simulink model "TestPDURacks"  (R2025b)
settings: Solver=daessc  StartTime=0.0  StopTime=1200  MaxStep=1  RelTol=1e-3  AbsTol=1e-3
libraries: nesl_utility x5, fl_lib x4, datacenterCompositeLib x1
settings Model: Creator=vikrants  LastModifiedBy=vikrants
settings SolverCC: AutoScaleAbsTol=off  AlgebraicLoopSolver=TrustRegion  MaxZcPerStep=1.0
settings DebuggingCC: UnconnectedInputMsg=warning  UnconnectedOutputMsg=warning  UnconnectedLineMsg=warning  SymbolicDimsDataTypeCodeGenerationDiagnostic=none
settings ModelReferenceCC: EnableRefExpFcnMdlSchedulingChecks=on
settings SFSimCC: CustomCodeUndefinedFunction=UseInterfaceOnly
settings RTWCC: GPUComputeCapability=3.5  DLArmComputeVersion=19.05
settings SimscapeCC: SimscapeLogType=all  SimscapeLogSimulationStatistics=on  SimscapeLogDataHistory=10000.0

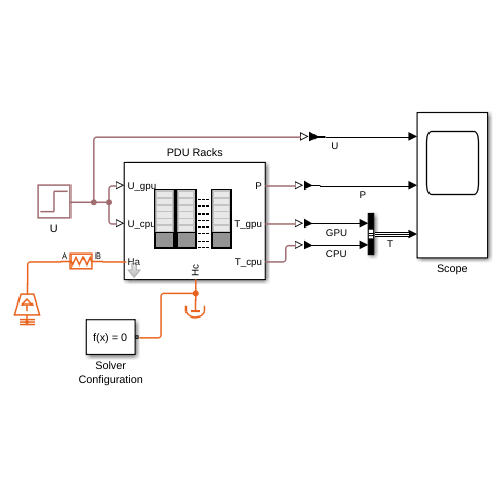
[thumbnail: Simulink's stored preview of the top-level diagram]
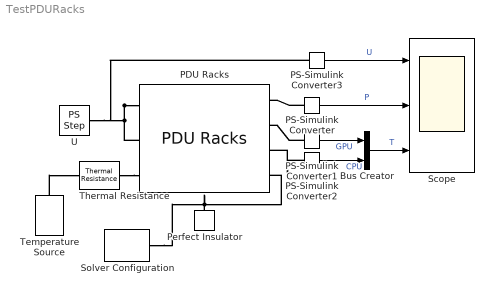
== system TestPDURacks ==
  Bus Creator : BusCreator  Inputs=2
  PDU Racks : datacenterCompositeLib/PDU Racks  nTrays=6  nRacks=4  trayMass=5  trayCp=2000  trayThermalR=0.1  nGPU=1  gpuTDPperDie=1200  gpuIdlePower=300  gpuHBMpower=80  gpuExponent=1.4  gpuHBMutil=0.7  gpuLeakage=1.5  gpuNominalDieT=350  gpuDieThermalC=50  gpuHeatSinkR=0.15  gpuSurfArea=0.01  gpuAmbientR=0.5  nCPU=1  cpuTDPperSocket=350  cpuIdlePower=80  cpuExponent=1.1  cpuLeakage=1.5  cpuNominalDieT=350  cpuDieThermalC=50  cpuHeatSinkR=0.15  cpuSurfArea=0.01  cpuAmbientR=0.5  initialT=350  htc=10
  PS-Simulink Converter{,1..3} (4 alike) : nesl_utility/PS-Simulink Converter  PhysicalDomain=network_engine_domain  SubClassName=ps_output  LeftPortType=input  RightPortType=output  PseudoPeriodic=off  Frequencies=[]  VectorFormat=inherit  Unit=inherit  AffineConversion=off
  Perfect Insulator : fl_lib/Thermal/Thermal Elements/Perfect Insulator  T_specify=off  T_priority=None  T=293.15 K  T_nominal_specify=off  T_nominal_value=1  T_nominal_unit=K
  Scope : Scope  NumInputPorts=3
      settings: ActiveDisplayYMinimum=0.15000000000000002  ActiveDisplayYMaximum=0.64999999999999991
  Solver Configuration : nesl_utility/Solver Configuration  PhysicalDomain=network_engine_domain  SubClassName=solver  LeftPortType=input  RightPortType=generic  Tones=[]  Harmonics=[]  SimulateNoise=off  Profile=off  UseLocalSampling=off  EnableSwitchedLinearOptims=on  FrequencyDomain=off  UseCCode=off  RelTol=0.001  AbsTol=1e-06  MinStep=1e-09  ToWorkspace=off  RevertToSquareIcSolve=off  NumHomotopyIterations=100  PhasorMode=off  PhasorModeNumHarmonics=1  ConsistencySolver=NEWTON_XTOL_AFTER_FTOL  IndexReductionMethod=DerivativeReplacement  DoDC=off  ResidualTolerance=1e-09  ConsistencyTolSource=GLOBAL  ConsistencyAbsTol=0.001  ConsistencyRelTol=0.001  ConsistencyTolFactor=0.001  UseLocalSolver=off  LocalSolverChoice=NE_BACKWARD_EULER_ADVANCER  ResolveIndetEquations=on  FunctionEvalNumThread=1  LocalSolverSampleTime=0.001  DoFixedCost=off  MaxNonlinIter=3  MaxModeIter=2  ComputeImpulses=off  ImpulseIterations=2  LinearAlgebra=auto  LinearAlgebraNumThread=0  EquationFormulation=NE_TIME_EF  DelaysMemoryBudget=1024  AutomaticFiltering=on  FilteringTimeConstant=0.001  PartitionStorageMethod=AS_NEEDED  PartitionMemoryBudget=1024  PartitionMethod=ROBUST  MultibodyUseLocalSolver=off  MultibodyLocalSolverChoice=ODE1  MultibodyLocalSolverSampleTime=0.001
  Temperature Source : fl_lib/Thermal/Thermal Sources/Temperature Source  temperature=293.15 K
  Thermal Resistance : fl_lib/Thermal/Thermal Elements/Thermal Resistance  resistance=1e-2 K/W  T_specify=off  T_priority=None  T=0 K  T_nominal_specify=off  T_nominal_value=1  T_nominal_unit=K  Q_specify=off  Q_priority=None  Q=0 W  Q_nominal_specify=off  Q_nominal_value=1  Q_nominal_unit=W
  U : fl_lib/Physical Signals/Sources/PS Step  step_time=600 s  initial_value=0.6  final_value=0.2
  wires:
  PS-Simulink Converter/1 -> Scope/2  "P"
  PS-Simulink Converter1/1 -> Bus Creator/1  "GPU"
  PS-Simulink Converter2/1 -> Bus Creator/2  "CPU"
  Bus Creator/1 -> Scope/3  "T"
  PS-Simulink Converter3/1 -> Scope/1  "U"
  connections:
  PDU Racks/LConn1 -- PS-Simulink Converter3/LConn1 -- U/RConn1 -- PDU Racks/LConn2
  Thermal Resistance/RConn1 -- PDU Racks/LConn3
  Temperature Source/LConn1 -- Thermal Resistance/LConn1
  Perfect Insulator/LConn1 -- Solver Configuration/RConn1 -- PDU Racks/RConn4
  PS-Simulink Converter/LConn1 -- PDU Racks/RConn1
  PS-Simulink Converter1/LConn1 -- PDU Racks/RConn2
  PS-Simulink Converter2/LConn1 -- PDU Racks/RConn3
